simulink model "lab3_fs_lqr_11_sim"  (R2024b)
settings: Solver=VariableStepAuto  StartTime=0.0  StopTime=20  FixedStep=1e-5  RelTol=1e-3
undefined symbols (not defined in the file or in its folder): beam, degs2rpm, deltaSS, drv, FS_LQR_A_q, FS_LQR_A_q_Ke_1, FS_LQR_A_q_Ki, FS_LQR_A_q_Nue, FS_LQR_A_q_Nxe, FS_LQR_B_q, FS_LQR_I, FS_LQR_zero, gbox, joint, lab3, mot, rads2rpm, rpm2rads, sens, step_amplitude, Ts, wcSS
settings Model: Creator=andre  LastModifiedBy=andre

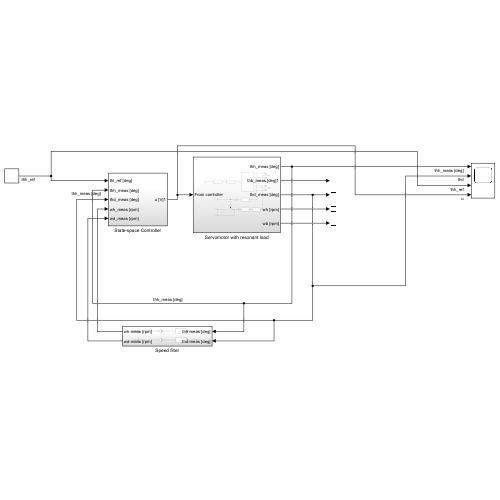
[thumbnail: Simulink's stored preview of the top-level diagram]
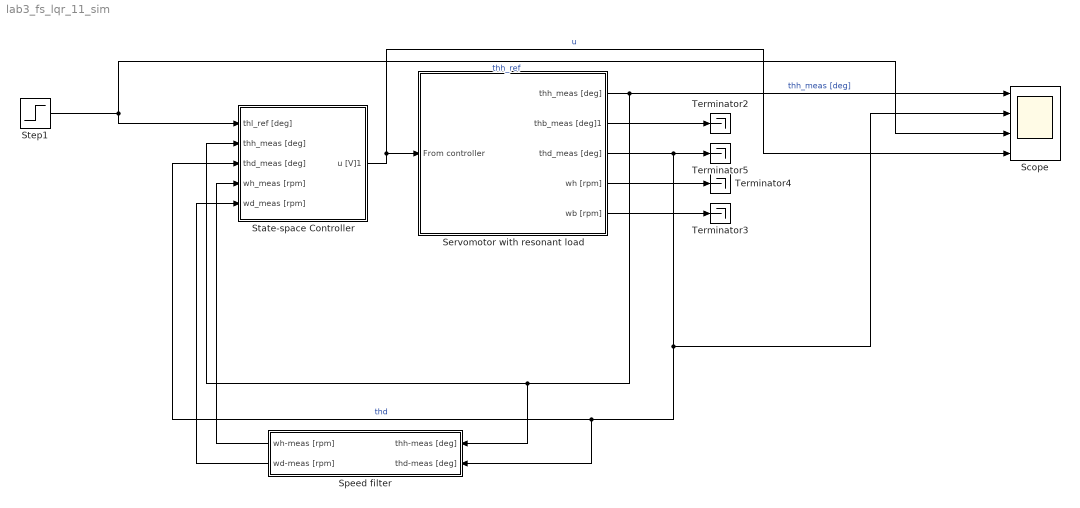
== system lab3_fs_lqr_11_sim ==
  Scope : Scope  NumInputPorts=4
  Servomotor with resonant load : Subsystem
  Speed filter : Subsystem
  State-space Controller : Subsystem
  Step1 : Step  Time=0  After=step_amplitude  SampleTime=0
  Terminator{2..5} (4 alike) : Terminator
  wires:
  Step1/1 -> Scope/3, State-space Controller/1(thl_ref [deg])  "thh_ref"
  Servomotor with resonant load/2(thb_meas [deg]1) -> Terminator2/1
  Servomotor with resonant load/1(thh_meas [deg]) -> Speed filter/1(thh-meas [deg]), State-space Controller/2(thh_meas [deg]), Scope/1  "thh_meas [deg]"
  Servomotor with resonant load/5(wb [rpm]) -> Terminator3/1
  Servomotor with resonant load/3(thd_meas [deg]) -> Speed filter/2(thd-meas [deg]), State-space Controller/3(thd_meas [deg]), Scope/2, Terminator5/1  "thd"
  Servomotor with resonant load/4(wh [rpm]) -> Terminator4/1
  State-space Controller/1(u [V]1) -> Scope/4, Servomotor with resonant load/1(From controller)  "u"
  Speed filter/1(wh-meas [rpm]) -> State-space Controller/4(wh_meas [rpm])
  Speed filter/2(wd-meas [rpm]) -> State-space Controller/5(wd_meas [rpm])

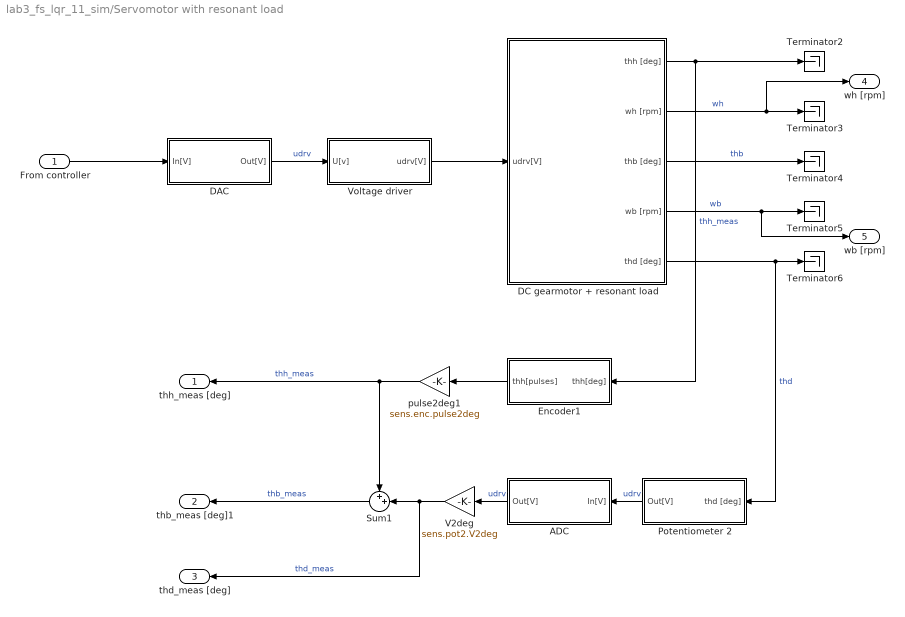
== system lab3_fs_lqr_11_sim/Servomotor with resonant load ==
  From controller : Inport
  ADC : Subsystem
  DAC : Subsystem
  DC gearmotor + resonant load : Subsystem
  Encoder1 : Subsystem
  Potentiometer 2 : Subsystem
  Sum1 : Sum  Inputs=++|
  Terminator{2..6} (5 alike) : Terminator
  V2deg : Gain  Gain=sens.pot2.V2deg
  Voltage driver : Subsystem
  pulse2deg1 : Gain  Gain=sens.enc.pulse2deg
  thh_meas [deg] : Outport
  thb_meas [deg]1 : Outport  Port=2
  thd_meas [deg] : Outport  Port=3
  wh [rpm] : Outport  Port=4
  wb [rpm] : Outport  Port=5
  wires:
  DC gearmotor + resonant load/5(thd [deg]) -> Potentiometer 2/1(thd [deg]), Terminator6/1  "thd"
  Sum1/1 -> thb_meas [deg]1/1  "thb_meas"
  DAC/1(Out[V]) -> Voltage driver/1(U[v])  "udrv"
  Voltage driver/1(udrv[V]) -> DC gearmotor + resonant load/1(udrv[V])
  Potentiometer 2/1(Out[V]) -> ADC/1(In[V])  "udrv"
  ADC/1(Out[V]) -> V2deg/1  "udrv"
  From controller/1 -> DAC/1(In[V])
  DC gearmotor + resonant load/3(thb [deg]) -> Terminator4/1  "thb"
  DC gearmotor + resonant load/4(wb [rpm]) -> wb [rpm]/1, Terminator5/1  "wb"
  DC gearmotor + resonant load/2(wh [rpm]) -> wh [rpm]/1, Terminator3/1  "wh"
  DC gearmotor + resonant load/1(thh [deg]) -> Encoder1/1(thh[deg]), Terminator2/1  "thh_meas"
  V2deg/1 -> thd_meas [deg]/1, Sum1/2  "thd_meas"
  Encoder1/1(thh[pulses]) -> pulse2deg1/1
  pulse2deg1/1 -> Sum1/1, thh_meas [deg]/1  "thh_meas"

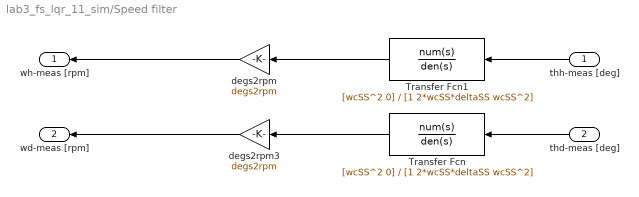
== system lab3_fs_lqr_11_sim/Speed filter ==
  thh-meas [deg] : Inport
  thd-meas [deg] : Inport  Port=2
  Transfer Fcn : TransferFcn  Numerator=[wcSS^2 0]  Denominator=[1 2*wcSS*deltaSS wcSS^2]
  Transfer Fcn1 : TransferFcn  Numerator=[wcSS^2 0]  Denominator=[1 2*wcSS*deltaSS wcSS^2]
  degs2rpm : Gain  Gain=degs2rpm
  degs2rpm3 : Gain  Gain=degs2rpm
  wh-meas [rpm] : Outport
  wd-meas [rpm] : Outport  Port=2
  wires:
  degs2rpm/1 -> wh-meas [rpm]/1
  Transfer Fcn1/1 -> degs2rpm/1
  degs2rpm3/1 -> wd-meas [rpm]/1
  thh-meas [deg]/1 -> Transfer Fcn1/1
  thd-meas [deg]/1 -> Transfer Fcn/1
  Transfer Fcn/1 -> degs2rpm3/1

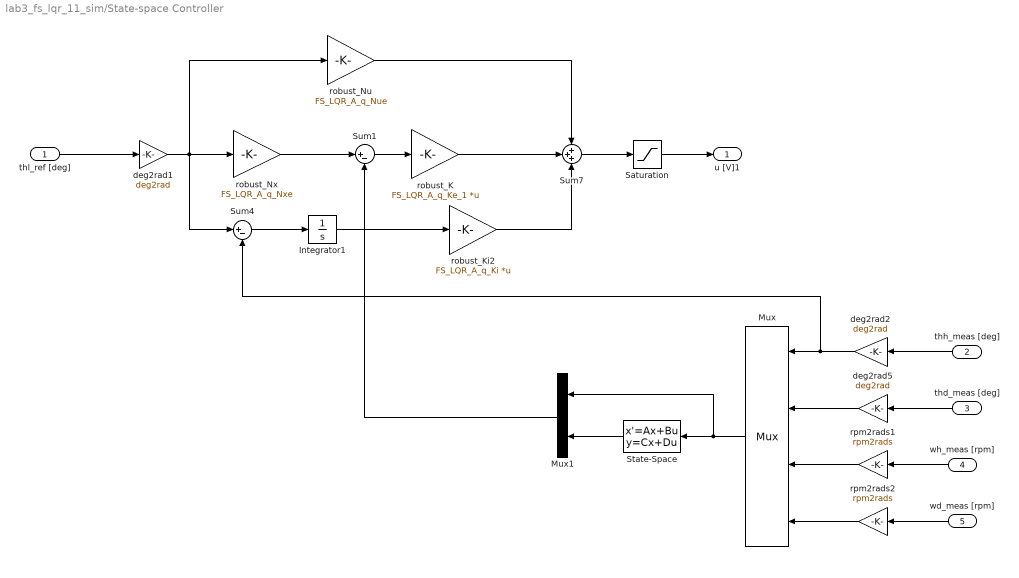
== system lab3_fs_lqr_11_sim/State-space Controller ==
  thl_ref [deg] : Inport
  thh_meas [deg] : Inport  Port=2
  thd_meas [deg] : Inport  Port=3
  wh_meas [rpm] : Inport  Port=4
  wd_meas [rpm] : Inport  Port=5
  Integrator1 : Integrator
  Mux : Mux
      settings: DisplayOption=signals
  Mux1 : Mux  Inputs=2
  Saturation : Saturate  UpperLimit=10  LowerLimit=-10
  State-Space : StateSpace  A=FS_LQR_A_q  B=FS_LQR_B_q  C=FS_LQR_I  D=FS_LQR_zero  InitialCondition=0
  Sum1 : Sum  Inputs=|+-
  Sum4 : Sum  Inputs=|+-
  Sum7 : Sum  Inputs=+++
  deg2rad1 : Gain  Gain=deg2rad
  deg2rad2 : Gain  Gain=deg2rad
  deg2rad5 : Gain  Gain=deg2rad
  robust_K : Gain  Gain=FS_LQR_A_q_Ke_1  Multiplication=Matrix(K*u)
  robust_Ki2 : Gain  Gain=FS_LQR_A_q_Ki  Multiplication=Matrix(K*u)
  robust_Nu : Gain  Gain=FS_LQR_A_q_Nue
  robust_Nx : Gain  Gain=FS_LQR_A_q_Nxe
  rpm2rads1 : Gain  Gain=rpm2rads
  rpm2rads2 : Gain  Gain=rpm2rads
  u [V]1 : Outport
  wires:
  Saturation/1 -> u [V]1/1
  deg2rad2/1 -> Sum4/2, Mux/1
  thl_ref [deg]/1 -> deg2rad1/1
  deg2rad1/1 -> Sum4/1, robust_Nu/1, robust_Nx/1
  Sum7/1 -> Saturation/1
  thh_meas [deg]/1 -> deg2rad2/1
  Sum1/1 -> robust_K/1
  deg2rad5/1 -> Mux/2
  robust_Nu/1 -> Sum7/1
  thd_meas [deg]/1 -> deg2rad5/1
  robust_Nx/1 -> Sum1/1
  wh_meas [rpm]/1 -> rpm2rads1/1
  rpm2rads1/1 -> Mux/3
  rpm2rads2/1 -> Mux/4
  wd_meas [rpm]/1 -> rpm2rads2/1
  robust_K/1 -> Sum7/2
  Mux/1 -> Mux1/1, State-Space/1
  State-Space/1 -> Mux1/2
  Mux1/1 -> Sum1/2
  robust_Ki2/1 -> Sum7/3
  Sum4/1 -> Integrator1/1
  Integrator1/1 -> robust_Ki2/1

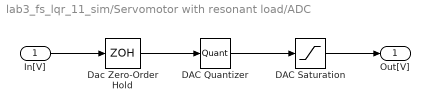
== system lab3_fs_lqr_11_sim/Servomotor with resonant load/ADC ==
  In[V] : Inport
  DAC Quantizer : Quantizer  QuantizationInterval=20/(2^16-1)
  DAC Saturation : Saturate  UpperLimit=10  LowerLimit=-10
  Dac Zero-Order Hold : ZeroOrderHold  SampleTime=Ts
  Out[V] : Outport
  wires:
  In[V]/1 -> Dac Zero-Order Hold/1
  DAC Saturation/1 -> Out[V]/1
  DAC Quantizer/1 -> DAC Saturation/1
  Dac Zero-Order Hold/1 -> DAC Quantizer/1

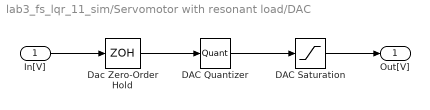
== system lab3_fs_lqr_11_sim/Servomotor with resonant load/DAC ==
  In[V] : Inport
  DAC Quantizer : Quantizer  QuantizationInterval=20/(2^16-1)
  DAC Saturation : Saturate  UpperLimit=10  LowerLimit=-10
  Dac Zero-Order Hold : ZeroOrderHold  SampleTime=Ts
  Out[V] : Outport
  wires:
  In[V]/1 -> Dac Zero-Order Hold/1
  DAC Saturation/1 -> Out[V]/1
  DAC Quantizer/1 -> DAC Saturation/1
  Dac Zero-Order Hold/1 -> DAC Quantizer/1

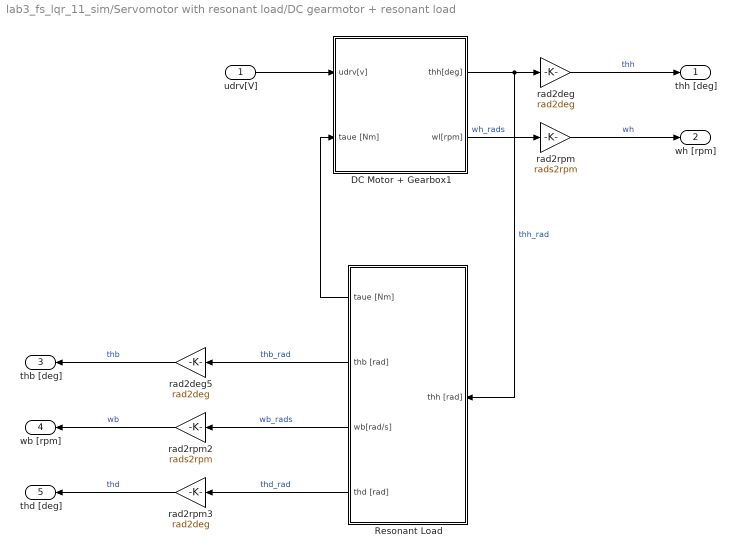
== system lab3_fs_lqr_11_sim/Servomotor with resonant load/DC gearmotor + resonant load ==
  udrv[V] : Inport
  DC Motor + Gearbox1 : Subsystem
  Resonant Load : Subsystem
  rad2deg : Gain  Gain=rad2deg
  rad2deg5 : Gain  Gain=rad2deg
  rad2rpm : Gain  Gain=rads2rpm
  rad2rpm2 : Gain  Gain=rads2rpm
  rad2rpm3 : Gain  Gain=rad2deg
  thh [deg] : Outport
  wh [rpm] : Outport  Port=2
  thb [deg] : Outport  Port=3
  wb [rpm] : Outport  Port=4
  thd [deg] : Outport  Port=5
  wires:
  rad2deg5/1 -> thb [deg]/1  "thb"
  udrv[V]/1 -> DC Motor + Gearbox1/1(udrv[v])
  DC Motor + Gearbox1/2(wl[rpm]) -> rad2rpm/1  "wh_rads"
  rad2rpm/1 -> wh [rpm]/1  "wh"
  Resonant Load/3(wb[rad/s]) -> rad2rpm2/1  "wb_rads"
  rad2rpm3/1 -> thd [deg]/1  "thd"
  DC Motor + Gearbox1/1(thh[deg]) -> Resonant Load/1(thh [rad]), rad2deg/1  "thh_rad"
  Resonant Load/1(taue [Nm]) -> DC Motor + Gearbox1/2(taue [Nm])
  rad2rpm2/1 -> wb [rpm]/1  "wb"
  rad2deg/1 -> thh [deg]/1  "thh"
  Resonant Load/4(thd [rad]) -> rad2rpm3/1  "thd_rad"
  Resonant Load/2(thb [rad]) -> rad2deg5/1  "thb_rad"

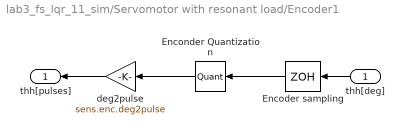
== system lab3_fs_lqr_11_sim/Servomotor with resonant load/Encoder1 ==
  thh[deg] : Inport
  Encoder sampling : ZeroOrderHold  SampleTime=Ts
  Enconder Quantization : Quantizer  QuantizationInterval=sens.enc.pulse2deg
  deg2pulse : Gain  Gain=sens.enc.deg2pulse
  thh[pulses] : Outport
  wires:
  thh[deg]/1 -> Encoder sampling/1
  Enconder Quantization/1 -> deg2pulse/1
  deg2pulse/1 -> thh[pulses]/1
  Encoder sampling/1 -> Enconder Quantization/1

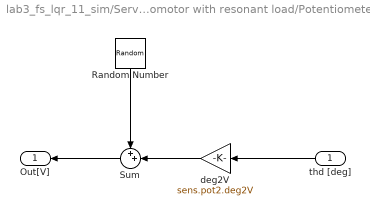
== system lab3_fs_lqr_11_sim/Servomotor with resonant load/Potentiometer 2 ==
  thd [deg] : Inport
  Random Number : RandomNumber  Variance=sens.pot2.noise.var  SampleTime=Ts
  Sum : Sum  Inputs=++|
  deg2V : Gain  Gain=sens.pot2.deg2V
  Out[V] : Outport
  wires:
  Random Number/1 -> Sum/1
  deg2V/1 -> Sum/2
  thd [deg]/1 -> deg2V/1
  Sum/1 -> Out[V]/1

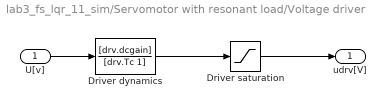
== system lab3_fs_lqr_11_sim/Servomotor with resonant load/Voltage driver ==
  U[v] : Inport
  Driver dynamics : TransferFcn  Numerator=[drv.dcgain]  Denominator=[drv.Tc 1]
  Driver saturation : Saturate  UpperLimit=12  LowerLimit=-12
  udrv[V] : Outport
  wires:
  U[v]/1 -> Driver dynamics/1
  Driver dynamics/1 -> Driver saturation/1
  Driver saturation/1 -> udrv[V]/1

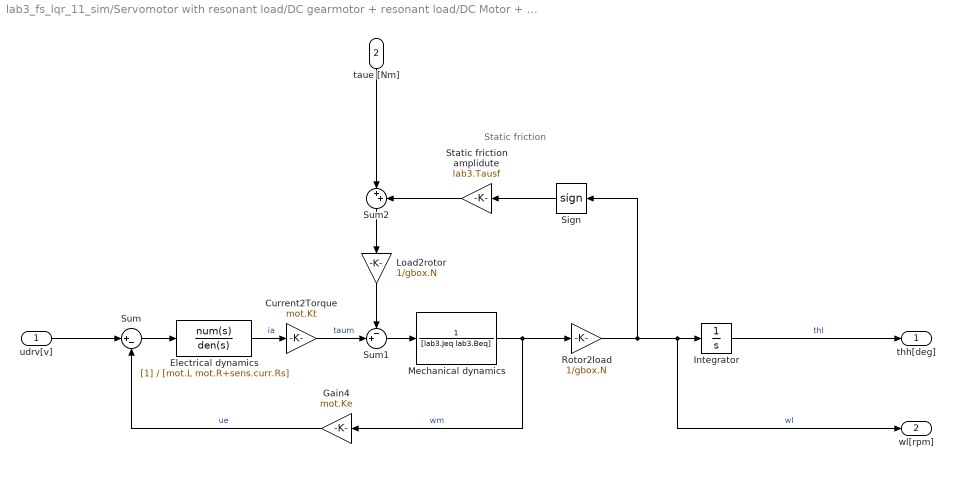
== system lab3_fs_lqr_11_sim/Servomotor with resonant load/DC gearmotor + resonant load/DC Motor + Gearbox1 ==
  note: Static friction
  udrv[v] : Inport
  taue [Nm] : Inport  Port=2
  " Sign" : Signum  ZeroCross=off
  Current2Torque : Gain  Gain=mot.Kt
  Electrical dynamics : TransferFcn  Denominator=[mot.L mot.R+sens.curr.Rs]
  Gain4 : Gain  Gain=mot.Ke
  Integrator : Integrator
  Load2rotor : Gain  Gain=1/gbox.N
  Mechanical dynamics : TransferFcn  Denominator=[lab3.Jeq lab3.Beq]
  Rotor2load : Gain  Gain=1/gbox.N
  Static friction amplidute : Gain  Gain=lab3.Tausf
  Sum : Sum  Inputs=|+-
  Sum1 : Sum  Inputs=-+|
  Sum2 : Sum  Inputs=|++
  thh[deg] : Outport
  wl[rpm] : Outport  Port=2
  wires:
  udrv[v]/1 -> Sum/1
  Sum/1 -> Electrical dynamics/1
  Electrical dynamics/1 -> Current2Torque/1  "ia"
  Current2Torque/1 -> Sum1/2  "taum"
  Load2rotor/1 -> Sum1/1
  " Sign"/1 -> Static friction amplidute/1
  Sum1/1 -> Mechanical dynamics/1
  Mechanical dynamics/1 -> Gain4/1, Rotor2load/1  "wm"
  Gain4/1 -> Sum/2  "ue"
  Integrator/1 -> thh[deg]/1  "thl"
  Rotor2load/1 -> " Sign"/1, wl[rpm]/1, Integrator/1  "wl"
  Sum2/1 -> Load2rotor/1
  Static friction amplidute/1 -> Sum2/2
  taue [Nm]/1 -> Sum2/1

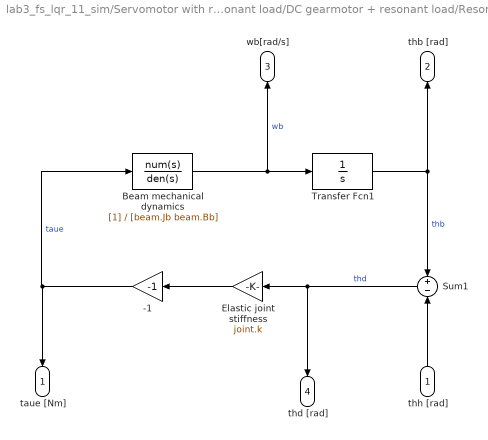
== system lab3_fs_lqr_11_sim/Servomotor with resonant load/DC gearmotor + resonant load/Resonant Load ==
  thh [rad] : Inport
  -1 : Gain  Gain=-1
  Beam mechanical dynamics : TransferFcn  Denominator=[beam.Jb beam.Bb]
  Elastic joint stiffness : Gain  Gain=joint.k
  Sum1 : Sum  Inputs=+|-
  Transfer Fcn1 : TransferFcn  Denominator=[1 0]
  taue [Nm] : Outport
  thb [rad] : Outport  Port=2
  wb[rad/s] : Outport  Port=3
  thd [rad] : Outport  Port=4
  wires:
  -1/1 -> taue [Nm]/1, Beam mechanical dynamics/1  "taue"
  Transfer Fcn1/1 -> thb [rad]/1, Sum1/1  "thb"
  Beam mechanical dynamics/1 -> wb[rad/s]/1, Transfer Fcn1/1  "wb"
  Elastic joint stiffness/1 -> -1/1
  thh [rad]/1 -> Sum1/2
  Sum1/1 -> thd [rad]/1, Elastic joint stiffness/1  "thd"
